simulink library "TotalCurrentCalculator"  (R2016b)
settings: Solver=VariableStepAuto  StartTime=0.0  StopTime=10.0  RelTol=1e-3
settings Model: Creator=Marc  LastModifiedBy=Marc

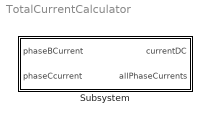
== system TotalCurrentCalculator ==
  Subsystem : Subsystem

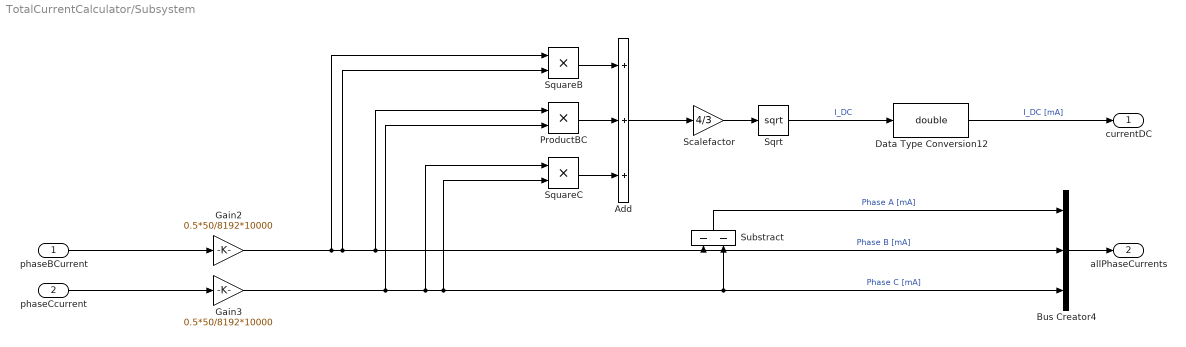
== system TotalCurrentCalculator/Subsystem ==
  phaseBCurrent : Inport  RequirementInfo={} %GIDa_e03d0c51_369a_4821_bfb5_259e526884e5
  phaseCcurrent : Inport  RequirementInfo={} %GIDa_e8a821eb_a83f_4f9e_b7b7_cfda67aa15b0  Port=2
  Add : Sum  RequirementInfo={} %GIDa_77bc119f_5099_4a80_bd0a_02fd7cd69863  Inputs=+++
  Bus Creator4 : BusCreator  RequirementInfo={} %GIDa_954082df_8983_48cc_898f_af4c8ee19079  Inputs=3
  Data Type Conversion12 : DataTypeConversion  RequirementInfo={} %GIDa_cb6c5b04_104d_4acd_94e6_2340374cb83a  OutDataTypeStr=double
  Gain2 : Gain  RequirementInfo={} %GIDa_8c589b43_9b4c_4ace_8ec7_38714aa2e449  Gain=0.5*50/8192*10000  OutDataTypeStr=double
  Gain3 : Gain  RequirementInfo={} %GIDa_8f165827_3543_4241_92c8_221dd33c48f7  Gain=0.5*50/8192*10000  OutDataTypeStr=double
  ProductBC : Product  RequirementInfo={} %GIDa_a8c560d2_9c7f_4274_b106_71780fc19769  Inputs=**
  Scalefactor : Gain  RequirementInfo={} %GIDa_2ea825b3_23ff_48c3_ac72_25f53d71a882  Gain=4/3
  Sqrt : Sqrt  RequirementInfo={} %GIDa_ebf708cb_e85b_433c_b2e0_ecc379ad8e86  SaturateOnIntegerOverflow=on
  SquareB : Product  RequirementInfo={} %GIDa_765bdec5_e42b_4889_82c8_002ff8ad8998  Inputs=**
  SquareC : Product  RequirementInfo={} %GIDa_c32a5f42_5294_4eaa_a3f1_1e34c0cbd870  Inputs=**
  Substract : Sum  RequirementInfo={} %GIDa_d5c2a15d_fb19_4909_88a4_7d45c4022f81  Inputs=--  OutDataTypeStr=double
  currentDC : Outport  RequirementInfo={} %GIDa_8f1a2852_eae9_4105_a27e_8c76e92028e7
  allPhaseCurrents : Outport  RequirementInfo={} %GIDa_79eacddf_537b_4404_900a_366b6f655d4e  Port=2
  wires:
  Bus Creator4/1 -> allPhaseCurrents/1
  Data Type Conversion12/1 -> currentDC/1  "I_DC [mA]"
  Substract/1 -> Bus Creator4/1  "Phase A [mA]"
  phaseCcurrent/1 -> Gain3/1
  phaseBCurrent/1 -> Gain2/1
  Gain2/1 -> SquareB/1, SquareB/2, ProductBC/1, Bus Creator4/2, Substract/1  "Phase B [mA]"
  Gain3/1 -> ProductBC/2, SquareC/1, SquareC/2, Bus Creator4/3, Substract/2  "Phase C [mA]"
  SquareB/1 -> Add/1
  Add/1 -> Scalefactor/1
  Sqrt/1 -> Data Type Conversion12/1  "I_DC"
  ProductBC/1 -> Add/2
  SquareC/1 -> Add/3
  Scalefactor/1 -> Sqrt/1
